simulink model "With_Hand_Real_Control_Cascaded"  (R2021a)
settings: Solver=FixedStepAuto  StartTime=0.0  StopTime=150  FixedStep=0.05  RelTol=1e-3  EnableMultiTasking=on
undefined symbols (not defined in the file or in its folder): sigbuilder_block
libraries: arduinolib x3, simulink x1, arduinosensorlib x1
PreSaveFcn:
  | set_param(gcs, 'Location',[35 56 895 650])
settings Model: ModifiedByFormat=The MathWorks Inc.  SimulationMode=external  SILPILModeSetting=veronly  ExtModeTrigDuration=2  Creator=The MathWorks Inc.  LastModifiedBy=The MathWorks Inc.
settings SolverCC: AlgebraicLoopSolver=TrustRegion
settings DataIOCC: LimitDataPoints=on  SaveFormat=Array  ReturnWorkspaceOutputs=off
settings OptimizationCC: LifeSpan=Inf  MaxStackSize=64
settings DebuggingCC: UnderspecifiedInitializationDetection=Classic  MergeDetectMultiDrivingBlocksExec=none  AllowSymbolicDim=off  SFUnexpectedBacktrackingDiag=warning  SFNoUnconditionalDefaultTransitionDiag=warning  SFMachineParentedDataDiag=warning  ArithmeticOperatorsInVariantConditions=warning
settings HardwareCC: ProdBitPerInt=16  ProdBitPerPointer=16  ProdBitPerSizeT=16  ProdBitPerPtrDiffT=16  ProdLargestAtomicFloat=None  ProdWordSize=8  ProdHWDeviceType=Atmel->AVR
settings ModelReferenceCC: PropagateSignalLabelsOutOfModel=off
settings SFSimCC: SimUseLocalCustomCode=off  CustomCodeUndefinedFunction=UseInterfaceOnly
settings RTWCC: SystemTargetFile=ert.tlc  HardwareBoard=Arduino Uno  TemplateMakefile=ert_default_tmf  RTWVerbose=off  RTWUseLocalCustomCode=off  Toolchain=Arduino AVR  BuildConfiguration=Faster Runs
settings CodeAppCC: StateflowObjectComments=on
settings ERTTargetCC: MultiwordLength=2048  ERTCustomFileBanners=off  SupportContinuousTime=on  SupportNonInlinedSFcns=on  SupportVariableSizeSignals=on  ModelStepFunctionPrototypeControlCompliant=off  ExtModeStaticAllocSize=250  ConvertIfToSwitch=off  SuppressUnreachableDefaultCases=off
settings ConfigComp: CovMetricSettings=dw  CovSaveCumulativeToWorkspaceVar=on  CovSaveSingleToWorkspaceVar=on  CovExternalEMLEnable=off  CovSFcnEnable=off

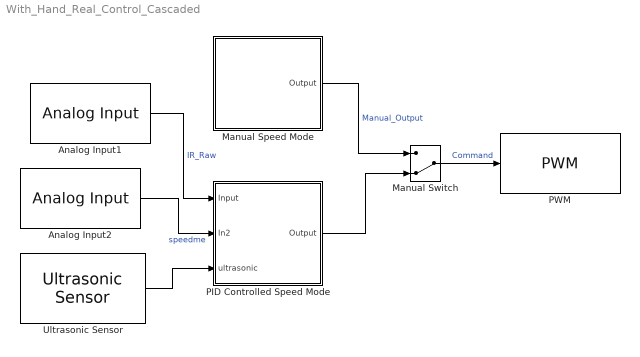
== system With_Hand_Real_Control_Cascaded ==
  Analog Input1 : arduinolib/Analog Input  pinNumber=1  ReadResultsOnly=off  ConversionTriggerSource=Software  ExternalTriggerType=uint32( 0 )  OutputDataType=uint16  EnableConversionCompleteNotify=off  EnableOuputStatus=off  SampleTime=1/20  blockPlatform=arduino
  Analog Input2 : arduinolib/Analog Input  pinNumber=4  ReadResultsOnly=off  ConversionTriggerSource=Software  ExternalTriggerType=uint32( 0 )  OutputDataType=uint16  EnableConversionCompleteNotify=off  EnableOuputStatus=off  SampleTime=1/20  blockPlatform=arduino
  Manual Speed Mode : Subsystem
  Manual Switch : ManualSwitch  CurrentSetting=0
  PID Controlled Speed Mode : Subsystem
  PWM : arduinolib/PWM  pinNumber=9  frequencyType=Default  desiredFrequency=490.2  achievableFrequency=490.2
  Ultrasonic Sensor : arduinosensorlib/Ultrasonic Sensor  NumSignalPins=2  TrigPin=3  EchoPin=5  SignalPin=3  SampleTime_=1/20  blockPlatform=ARDUINO
      settings: SourceProductBaseCode=ARDUINO
  wires:
  Manual Switch/1 -> PWM/1  "Command"
  Manual Speed Mode/1("Output ") -> Manual Switch/1  "Manual_Output"
  Analog Input1/1 -> PID Controlled Speed Mode/1(Input)  "IR_Raw"
  Analog Input2/1 -> PID Controlled Speed Mode/2(In2)  "speedme"
  PID Controlled Speed Mode/1(Output) -> Manual Switch/2
  Ultrasonic Sensor/1 -> PID Controlled Speed Mode/3(ultrasonic)

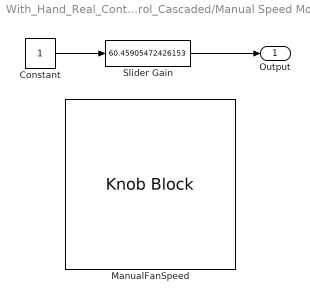
== system With_Hand_Real_Control_Cascaded/Manual Speed Mode ==
  Constant : Constant  OutDataTypeStr=single  SampleTime=0.05
  ManualFanSpeed : KnobBlock  ScaleMax=255
  Slider Gain : simulink/Math Operations/Slider Gain  gain=60.45905472426153  low=0  high=255
  "Output " : Outport
  wires:
  Slider Gain/1 -> "Output "/1
  Constant/1 -> Slider Gain/1

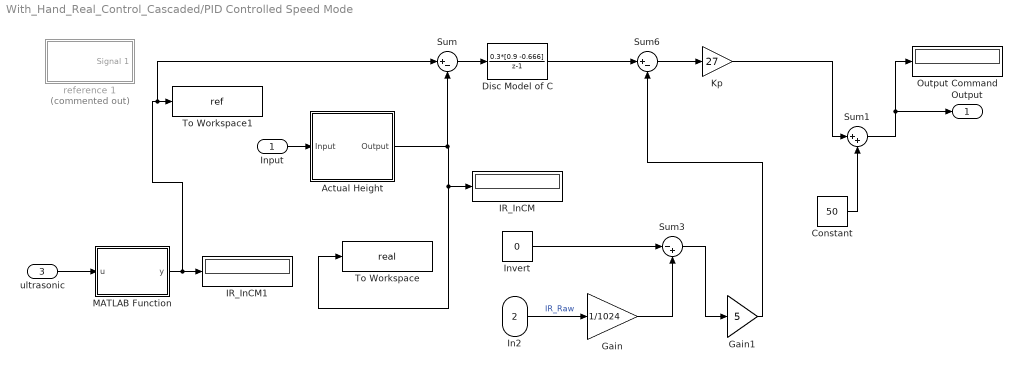
== system With_Hand_Real_Control_Cascaded/PID Controlled Speed Mode ==
  Input : Inport
  In2 : Inport  Port=2
  ultrasonic : Inport  Port=3
  Actual Height : Subsystem
  Constant : Constant  Value=50  SampleTime=0.05
  Disc Model of C : DiscreteTransferFcn  Numerator=0.3*[0.9 -0.666]  Denominator=[1 -1]  SampleTime=0.05
  Gain : Gain  Gain=1/1024
  Gain1 : Gain  Gain=5
  IR_InCM : Display
  IR_InCM1 : Display
  Invert : Constant  Value=0  OutDataTypeStr=single  SampleTime=0.05
  Kp : Gain  Gain=27
  MATLAB Function : MATLAB Function  TreatAsAtomicUnit=on
  "Output Command " : Display
  Sum : Sum  Inputs=|+-
  Sum1 : Sum  Inputs=|++
  Sum3 : Sum  Inputs=|-+
  Sum6 : Sum  Inputs=|+-
  To Workspace : ToWorkspace  VariableName=real  SampleTime=-1
      settings: Save2DSignal=2-D array (concatenate along first dimension)
  To Workspace1 : ToWorkspace  VariableName=ref  SampleTime=-1
      settings: Save2DSignal=2-D array (concatenate along first dimension)
  reference 1 : Subsystem  Tag=STV Subsys  Commented=on  LoadFcn=sigbuilder_block('load');  StartFcn=sigbuilder_block('start');  StopFcn=sigbuilder_block('stop');  ClipboardFcn=sigbuilder_block('clipboard');  mask(Sigbuilder block){tuvar=[0:10]}
      mask help: Simulink:masks:SigbuilderBlock_MD
      mask init:
      | if ~strcmp(get_param(bdroot(gcbh),'SimulationStatus'),'stopped') tuvar = sigbuilder_block('maskInit'); end
      settings: CopyFcn=sigbuilder_block('copy');  DeleteFcn=sigbuilder_block('delete');  ModelCloseFcn=sigbuilder_block('modelClose');  PreSaveFcn=sigbuilder_block('preSave');  PauseFcn=sigbuilder_block('pause');  ContinueFcn=sigbuilder_block('continue');  NameChangeFcn=sigbuilder_block('namechange');  OpenFcn=sigbuilder_block('open',[55.604 233.822 642.297 302.257 ]);  CloseFcn=sigbuilder_block('close');
      mask Display: plot(0, 0, 100, 100,[2, 2, 32, 32, 2], [68, 8, 8, 68, 68],[32, 2], [38, 38], [32, 19, 2],[53, 60, 44], [32, 17, 17, 2],[16, 16, 31, 31]);txt = getActiveGroup(gcbh);text(2, 100, txt,'verticalAlignment', 'top');
  Output : Outport
  wires:
  Input/1 -> Actual Height/1(Input)
  Actual Height/1(Output) -> To Workspace/1, IR_InCM/1, Sum/2
  Sum/1 -> Disc Model of C/1
  Disc Model of C/1 -> Sum6/1
  Sum6/1 -> Kp/1
  In2/1 -> Gain/1  "IR_Raw"
  Gain/1 -> Sum3/2
  Gain1/1 -> Sum6/2
  Kp/1 -> Sum1/1
  Constant/1 -> Sum1/2
  Sum1/1 -> "Output Command "/1, Output/1
  Invert/1 -> Sum3/1
  Sum3/1 -> Gain1/1
  ultrasonic/1 -> MATLAB Function/1(u)
  MATLAB Function/1(y) -> Sum/1, To Workspace1/1, IR_InCM1/1

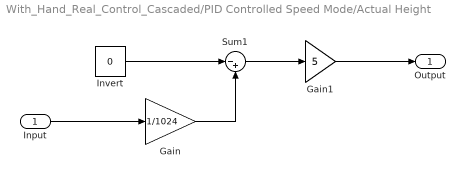
== system With_Hand_Real_Control_Cascaded/PID Controlled Speed Mode/Actual Height ==
  Input : Inport
  Gain : Gain  Gain=1/1024
  Gain1 : Gain  Gain=5
  Invert : Constant  Value=0  OutDataTypeStr=single  SampleTime=0.05
  Sum1 : Sum  Inputs=|-+
  Output : Outport
  wires:
  Input/1 -> Gain/1
  Invert/1 -> Sum1/1
  Gain/1 -> Sum1/2
  Sum1/1 -> Gain1/1
  Gain1/1 -> Output/1

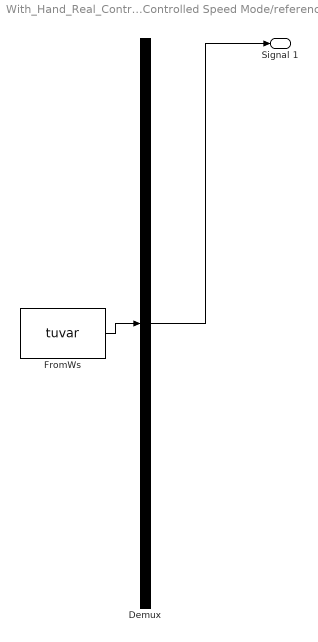
== system With_Hand_Real_Control_Cascaded/PID Controlled Speed Mode/reference 1 ==
  Demux : Demux  Tag=STV Demux  Outputs=1
      settings: DisplayOption=none
  FromWs : FromWorkspace  Tag=STV FromWs  VariableName=tuvar  SampleTime=0.05  ZeroCross=off  OutputAfterFinalValue=Setting to zero
      SigBuilderData=|
      | common.afterFinalStr = 'Set to zero'
      | common.sampleTime = '0.05'
      | dataSet.timeRange = [0 100]
      | dataSet.name = 'Group 1'
      | sbobj.Groups.Name = 'Group 1'
      | sbobj.Groups.Signals.Name = 'Signal 1'
      | sbobj.Groups.Signals.XData = [0 10.6 10.6 24.4 24.4 36 36 45.9 45.9 59.7 59.7 81.7 81.7 100]
      | sbobj.Groups.Signals.YData = [1.7 1.7 1.915 1.915 2.024 2.024 1.858 1.858 2.112 2.112 1.772 1.772 2.328 2.328]
      | sbobj.Groups.TimeRange = [0 100]
  Signal 1 : Outport  Tag=STV Outport
  wires:
  Demux/1 -> Signal 1/1
  FromWs/1 -> Demux/1

== matlab function With_Hand_Real_Control_Cascaded/PID Controlled Speed Mode/MATLAB Function ==
  data: u input; y output
function y = fcn(u)
p1 =   8.525e-06;
p2 =  -0.0004896 ;
p3 =     0.01173 ;
p4 =     -0.1058  ;
p5 =       1.228 ;
u = 100*u +8;
y = p1*u^4 + p2*u^3 + p3*u^2 + p4*u + p5;
if y>2.45
    y = 2.45;
end

end
